simulink model "busselector"  (Simulink 7.3)
settings: Solver=FixedStepDiscrete  StartTime=0.0  StopTime=10.0  FixedStep=1  RelTol=1e-3
settings Model: Creator=ksmyth  LastModifiedBy=hnine
settings DataIOCC: SaveFormat=Structure
settings OptimizationCC: InitFltsAndDblsToZero=on
settings DebuggingCC: SaveWithParameterizedLinksMsg=none
settings GRTTargetCC: TargetFcnLib=ansi_tfl_tmw.mat

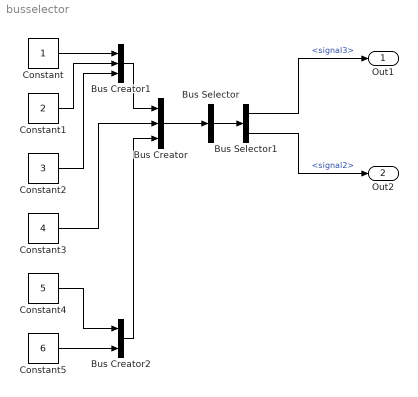
== system busselector ==
  Bus Creator : BusCreator  Inputs=3
  Bus Creator1 : BusCreator  Inputs=3
  Bus Creator2 : BusCreator  Inputs=2
  Bus Selector : BusSelector  OutputSignals=signal2,signal1,signal3  OutputAsBus=on
  Bus Selector1 : BusSelector  OutputSignals=signal3,signal2
  Constant : Constant  OutDataType=sfix(16)  OutScaling=2^0
  Constant1 : Constant  Value=2  OutDataType=sfix(16)  OutScaling=2^0
  Constant2 : Constant  Value=3  OutDataType=sfix(16)  OutScaling=2^0
  Constant3 : Constant  Value=4  OutDataType=sfix(16)  OutScaling=2^0
  Constant4 : Constant  Value=5  OutDataType=sfix(16)  OutScaling=2^0
  Constant5 : Constant  Value=6  OutDataType=sfix(16)  OutScaling=2^0
  Out1 : Outport  OutDataType=sfix(16)  OutScaling=2^0
  Out2 : Outport  Port=2  OutDataType=sfix(16)  OutScaling=2^0
  wires:
  Constant/1 -> Bus Creator1/1
  Constant1/1 -> Bus Creator1/2
  Constant2/1 -> Bus Creator1/3
  Constant3/1 -> Bus Creator/2
  Bus Creator/1 -> Bus Selector/1
  Bus Selector/1 -> Bus Selector1/1
  Constant4/1 -> Bus Creator2/1
  Bus Selector1/2 -> Out2/1  "<signal2>"
  Bus Selector1/1 -> Out1/1  "<signal3>"
  Bus Creator1/1 -> Bus Creator/1
  Constant5/1 -> Bus Creator2/2
  Bus Creator2/1 -> Bus Creator/3
